simulink model "Computer"  (R2023a)
settings: Solver=VariableStepDiscrete  StartTime=0.0  StopTime=inf  RelTol=1e-3  EnableMultiTasking=on
values from neighbouring files (symbols this model uses):
  RomCode = Preprocessor(RomCode, c)    [ROM.m]
undefined symbols (not defined in the file or in its folder): c, in, RomCodeBreakpoints, RomData, RomDataBreakpoints, UartDataRx, UartDataRx_Active
libraries: Miscellaneous x281, simulink_extras x66, Memory_Blocks_Lib x46, simulink x42, Word_Multiplexers_Lib x31, Decoders_Lib x30, Encoders_Lib x10, Counters_Lib x9, Bit_Multiplexers_Lib x8, Arithmetic_Operations_Lib x5, Bit_Demultiplexers_Lib x4, Garbage x1
(part 3 of 6)

== system Computer/<0x0000..0x0FFF> ==
  note: Address_Select
  b15 : Inport
  b14 : Inport  Port=2
  b13 : Inport  Port=3
  b12 : Inport  Port=4
  b11 : Inport  Port=5
  b10 : Inport  Port=6
  b09 : Inport  Port=7
  b08 : Inport  Port=8
  b07 : Inport  Port=9
  b06 : Inport  Port=10
  b05 : Inport  Port=11
  b04 : Inport  Port=12
  b03 : Inport  Port=13
  b02 : Inport  Port=14
  b01 : Inport  Port=15
  b00 : Inport  Port=16
  1 : Constant  OutDataTypeStr=boolean
  Logical Operator{10..12,17} (4 alike) : Logic  Operator=NOT  Inputs=1  IconShape=distinctive  AllPortsSameDT=off  OutDataTypeStr=boolean
  Logical Operator9 : Logic  Inputs=16  IconShape=distinctive  AllPortsSameDT=off  OutDataTypeStr=boolean
  Terminator{1..12} (12 alike) : Terminator
  Sel(1b) : Outport
  wires:
  Logical Operator9/1 -> Sel(1b)/1
  b13/1 -> Logical Operator12/1
  b15/1 -> Logical Operator10/1
  b14/1 -> Logical Operator11/1
  b12/1 -> Logical Operator17/1
  Logical Operator10/1 -> Logical Operator9/1
  Logical Operator11/1 -> Logical Operator9/2
  Logical Operator12/1 -> Logical Operator9/3
  Logical Operator17/1 -> Logical Operator9/4
  b00/1 -> Terminator12/1
  b11/1 -> Terminator9/1
  b10/1 -> Terminator8/1
  b09/1 -> Terminator7/1
  b08/1 -> Terminator6/1
  b07/1 -> Terminator5/1
  b06/1 -> Terminator4/1
  b05/1 -> Terminator3/1
  b04/1 -> Terminator1/1
  b03/1 -> Terminator2/1
  b02/1 -> Terminator10/1
  b01/1 -> Terminator11/1
  1/1 -> Logical Operator9/16, Logical Operator9/15, Logical Operator9/14, Logical Operator9/13, Logical Operator9/12, Logical Operator9/11, Logical Operator9/10, Logical Operator9/9, Logical Operator9/8, Logical Operator9/7, Logical Operator9/6, Logical Operator9/5

== system Computer/<0x1000..0x1FFF> ==
  note: Address_Select
  b15 : Inport
  b14 : Inport  Port=2
  b13 : Inport  Port=3
  b12 : Inport  Port=4
  b11 : Inport  Port=5
  b10 : Inport  Port=6
  b09 : Inport  Port=7
  b08 : Inport  Port=8
  b07 : Inport  Port=9
  b06 : Inport  Port=10
  b05 : Inport  Port=11
  b04 : Inport  Port=12
  b03 : Inport  Port=13
  b02 : Inport  Port=14
  b01 : Inport  Port=15
  b00 : Inport  Port=16
  1 : Constant  OutDataTypeStr=boolean
  Logical Operator10 : Logic  Operator=NOT  Inputs=1  IconShape=distinctive  AllPortsSameDT=off  OutDataTypeStr=boolean
  Logical Operator11 : Logic  Operator=NOT  Inputs=1  IconShape=distinctive  AllPortsSameDT=off  OutDataTypeStr=boolean
  Logical Operator12 : Logic  Operator=NOT  Inputs=1  IconShape=distinctive  AllPortsSameDT=off  OutDataTypeStr=boolean
  Logical Operator9 : Logic  Inputs=16  IconShape=distinctive  AllPortsSameDT=off  OutDataTypeStr=boolean
  Terminator{1..13} (13 alike) : Terminator
  Sel(1b) : Outport
  wires:
  Logical Operator9/1 -> Sel(1b)/1
  b13/1 -> Logical Operator12/1
  b15/1 -> Logical Operator10/1
  b14/1 -> Logical Operator11/1
  Logical Operator10/1 -> Logical Operator9/1
  Logical Operator11/1 -> Logical Operator9/2
  Logical Operator12/1 -> Logical Operator9/3
  b00/1 -> Terminator12/1
  b11/1 -> Terminator9/1
  b10/1 -> Terminator8/1
  b09/1 -> Terminator7/1
  b08/1 -> Terminator6/1
  b07/1 -> Terminator5/1
  b06/1 -> Terminator4/1
  b05/1 -> Terminator3/1
  b04/1 -> Terminator1/1
  b03/1 -> Terminator2/1
  b02/1 -> Terminator10/1
  b01/1 -> Terminator11/1
  1/1 -> Logical Operator9/16, Logical Operator9/15, Logical Operator9/14, Logical Operator9/13, Logical Operator9/12, Logical Operator9/11, Logical Operator9/10, Logical Operator9/9, Logical Operator9/8, Logical Operator9/7, Logical Operator9/6, Logical Operator9/4, Logical Operator9/5
  b12/1 -> Terminator13/1

== system Computer/<0x2000..0x23FF> ==
  note: Address_Select
  b15 : Inport
  b14 : Inport  Port=2
  b13 : Inport  Port=3
  b12 : Inport  Port=4
  b11 : Inport  Port=5
  b10 : Inport  Port=6
  b09 : Inport  Port=7
  b08 : Inport  Port=8
  b07 : Inport  Port=9
  b06 : Inport  Port=10
  b05 : Inport  Port=11
  b04 : Inport  Port=12
  b03 : Inport  Port=13
  b02 : Inport  Port=14
  b01 : Inport  Port=15
  b00 : Inport  Port=16
  1 : Constant  OutDataTypeStr=boolean
  Logical Operator{1,4..5,10..11} (5 alike) : Logic  Operator=NOT  Inputs=1  IconShape=distinctive  AllPortsSameDT=off  OutDataTypeStr=boolean
  Logical Operator9 : Logic  Inputs=16  IconShape=distinctive  AllPortsSameDT=off  OutDataTypeStr=boolean
  Terminator{1..7,10..12} (10 alike) : Terminator
  Sel(1b) : Outport
  wires:
  Logical Operator9/1 -> Sel(1b)/1
  b15/1 -> Logical Operator10/1
  b14/1 -> Logical Operator11/1
  Logical Operator10/1 -> Logical Operator9/1
  Logical Operator11/1 -> Logical Operator9/2
  b00/1 -> Terminator12/1
  b09/1 -> Terminator7/1
  b08/1 -> Terminator6/1
  b07/1 -> Terminator5/1
  b06/1 -> Terminator4/1
  b05/1 -> Terminator3/1
  b04/1 -> Terminator1/1
  b03/1 -> Terminator2/1
  b02/1 -> Terminator10/1
  b01/1 -> Terminator11/1
  1/1 -> Logical Operator9/16, Logical Operator9/15, Logical Operator9/14, Logical Operator9/13, Logical Operator9/12, Logical Operator9/11, Logical Operator9/10, Logical Operator9/9, Logical Operator9/8, Logical Operator9/7
  Logical Operator4/1 -> Logical Operator9/4
  Logical Operator5/1 -> Logical Operator9/6
  Logical Operator1/1 -> Logical Operator9/5
  b13/1 -> Logical Operator9/3
  b12/1 -> Logical Operator4/1
  b11/1 -> Logical Operator1/1
  b10/1 -> Logical Operator5/1

== system Computer/<0xFFF6..0xFFF6> ==
  note: Address_Select
  b15 : Inport
  b14 : Inport  Port=2
  b13 : Inport  Port=3
  b12 : Inport  Port=4
  b11 : Inport  Port=5
  b10 : Inport  Port=6
  b09 : Inport  Port=7
  b08 : Inport  Port=8
  b07 : Inport  Port=9
  b06 : Inport  Port=10
  b05 : Inport  Port=11
  b04 : Inport  Port=12
  b03 : Inport  Port=13
  b02 : Inport  Port=14
  b01 : Inport  Port=15
  b00 : Inport  Port=16
  Logical Operator17 : Logic  Operator=NOT  Inputs=1  IconShape=distinctive  AllPortsSameDT=off  OutDataTypeStr=boolean
  Logical Operator2 : Logic  Operator=NOT  Inputs=1  IconShape=distinctive  AllPortsSameDT=off  OutDataTypeStr=boolean
  Logical Operator9 : Logic  Inputs=16  IconShape=distinctive  AllPortsSameDT=off  OutDataTypeStr=boolean
  Sel(1b) : Outport
  wires:
  Logical Operator9/1 -> Sel(1b)/1
  b00/1 -> Logical Operator17/1
  Logical Operator17/1 -> Logical Operator9/16
  b11/1 -> Logical Operator9/5
  b10/1 -> Logical Operator9/6
  b09/1 -> Logical Operator9/7
  b08/1 -> Logical Operator9/8
  b07/1 -> Logical Operator9/9
  b06/1 -> Logical Operator9/10
  b05/1 -> Logical Operator9/11
  b04/1 -> Logical Operator9/12
  b02/1 -> Logical Operator9/14
  b01/1 -> Logical Operator9/15
  b12/1 -> Logical Operator9/4
  b13/1 -> Logical Operator9/3
  b14/1 -> Logical Operator9/2
  b15/1 -> Logical Operator9/1
  Logical Operator2/1 -> Logical Operator9/13
  b03/1 -> Logical Operator2/1

== system Computer/<0xFFF7..0xFFF7> ==
  note: Address_Select
  b15 : Inport
  b14 : Inport  Port=2
  b13 : Inport  Port=3
  b12 : Inport  Port=4
  b11 : Inport  Port=5
  b10 : Inport  Port=6
  b09 : Inport  Port=7
  b08 : Inport  Port=8
  b07 : Inport  Port=9
  b06 : Inport  Port=10
  b05 : Inport  Port=11
  b04 : Inport  Port=12
  b03 : Inport  Port=13
  b02 : Inport  Port=14
  b01 : Inport  Port=15
  b00 : Inport  Port=16
  Logical Operator5 : Logic  Operator=NOT  Inputs=1  IconShape=distinctive  AllPortsSameDT=off  OutDataTypeStr=boolean
  Logical Operator9 : Logic  Inputs=16  IconShape=distinctive  AllPortsSameDT=off  OutDataTypeStr=boolean
  Sel(1b) : Outport
  wires:
  Logical Operator9/1 -> Sel(1b)/1
  Logical Operator5/1 -> Logical Operator9/13
  b03/1 -> Logical Operator5/1
  b15/1 -> Logical Operator9/1
  b14/1 -> Logical Operator9/2
  b13/1 -> Logical Operator9/3
  b12/1 -> Logical Operator9/4
  b11/1 -> Logical Operator9/5
  b10/1 -> Logical Operator9/6
  b09/1 -> Logical Operator9/7
  b08/1 -> Logical Operator9/8
  b07/1 -> Logical Operator9/9
  b06/1 -> Logical Operator9/10
  b05/1 -> Logical Operator9/11
  b04/1 -> Logical Operator9/12
  b02/1 -> Logical Operator9/14
  b01/1 -> Logical Operator9/15
  b00/1 -> Logical Operator9/16

== system Computer/<0xFFF8..0xFFFD> ==
  note: Address_Select
  b15 : Inport
  b14 : Inport  Port=2
  b13 : Inport  Port=3
  b12 : Inport  Port=4
  b11 : Inport  Port=5
  b10 : Inport  Port=6
  b09 : Inport  Port=7
  b08 : Inport  Port=8
  b07 : Inport  Port=9
  b06 : Inport  Port=10
  b05 : Inport  Port=11
  b04 : Inport  Port=12
  b03 : Inport  Port=13
  b02 : Inport  Port=14
  b01 : Inport  Port=15
  b00 : Inport  Port=16
  1 : Constant  OutDataTypeStr=boolean
  Logical Operator9 : Logic  Inputs=16  IconShape=distinctive  AllPortsSameDT=off  OutDataTypeStr=boolean
  Terminator10 : Terminator
  Terminator11 : Terminator
  Terminator12 : Terminator
  Sel(1b) : Outport
  wires:
  Logical Operator9/1 -> Sel(1b)/1
  b13/1 -> Logical Operator9/3
  b15/1 -> Logical Operator9/1
  b14/1 -> Logical Operator9/2
  b00/1 -> Terminator12/1
  b11/1 -> Logical Operator9/5
  b10/1 -> Logical Operator9/6
  b09/1 -> Logical Operator9/7
  b08/1 -> Logical Operator9/8
  b07/1 -> Logical Operator9/9
  b06/1 -> Logical Operator9/10
  b05/1 -> Logical Operator9/11
  b04/1 -> Logical Operator9/12
  b03/1 -> Logical Operator9/13
  b02/1 -> Terminator10/1
  b01/1 -> Terminator11/1
  1/1 -> Logical Operator9/16, Logical Operator9/15, Logical Operator9/14
  b12/1 -> Logical Operator9/4

== system Computer/<0xFFF8..0xFFFD>1 ==
  note: Address_Select
  b15 : Inport
  b14 : Inport  Port=2
  b13 : Inport  Port=3
  b12 : Inport  Port=4
  b11 : Inport  Port=5
  b10 : Inport  Port=6
  b09 : Inport  Port=7
  b08 : Inport  Port=8
  b07 : Inport  Port=9
  b06 : Inport  Port=10
  b05 : Inport  Port=11
  b04 : Inport  Port=12
  b03 : Inport  Port=13
  b02 : Inport  Port=14
  b01 : Inport  Port=15
  b00 : Inport  Port=16
  1 : Constant  OutDataTypeStr=boolean
  Logical Operator9 : Logic  Inputs=16  IconShape=distinctive  AllPortsSameDT=off  OutDataTypeStr=boolean
  Terminator10 : Terminator
  Terminator11 : Terminator
  Terminator12 : Terminator
  Sel(1b) : Outport
  wires:
  Logical Operator9/1 -> Sel(1b)/1
  b13/1 -> Logical Operator9/3
  b15/1 -> Logical Operator9/1
  b14/1 -> Logical Operator9/2
  b00/1 -> Terminator12/1
  b11/1 -> Logical Operator9/5
  b10/1 -> Logical Operator9/6
  b09/1 -> Logical Operator9/7
  b08/1 -> Logical Operator9/8
  b07/1 -> Logical Operator9/9
  b06/1 -> Logical Operator9/10
  b05/1 -> Logical Operator9/11
  b04/1 -> Logical Operator9/12
  b03/1 -> Logical Operator9/13
  b02/1 -> Terminator10/1
  b01/1 -> Terminator11/1
  1/1 -> Logical Operator9/16, Logical Operator9/15, Logical Operator9/14
  b12/1 -> Logical Operator9/4

== system Computer/<0xFFFE..0xFFFE> ==
  note: Address_Select
  b15 : Inport
  b14 : Inport  Port=2
  b13 : Inport  Port=3
  b12 : Inport  Port=4
  b11 : Inport  Port=5
  b10 : Inport  Port=6
  b09 : Inport  Port=7
  b08 : Inport  Port=8
  b07 : Inport  Port=9
  b06 : Inport  Port=10
  b05 : Inport  Port=11
  b04 : Inport  Port=12
  b03 : Inport  Port=13
  b02 : Inport  Port=14
  b01 : Inport  Port=15
  b00 : Inport  Port=16
  Logical Operator17 : Logic  Operator=NOT  Inputs=1  IconShape=distinctive  AllPortsSameDT=off  OutDataTypeStr=boolean
  Logical Operator9 : Logic  Inputs=16  IconShape=distinctive  AllPortsSameDT=off  OutDataTypeStr=boolean
  Sel(1b) : Outport
  wires:
  Logical Operator9/1 -> Sel(1b)/1
  b00/1 -> Logical Operator17/1
  Logical Operator17/1 -> Logical Operator9/16
  b11/1 -> Logical Operator9/5
  b10/1 -> Logical Operator9/6
  b09/1 -> Logical Operator9/7
  b08/1 -> Logical Operator9/8
  b07/1 -> Logical Operator9/9
  b06/1 -> Logical Operator9/10
  b05/1 -> Logical Operator9/11
  b04/1 -> Logical Operator9/12
  b03/1 -> Logical Operator9/13
  b02/1 -> Logical Operator9/14
  b01/1 -> Logical Operator9/15
  b12/1 -> Logical Operator9/4
  b13/1 -> Logical Operator9/3
  b14/1 -> Logical Operator9/2
  b15/1 -> Logical Operator9/1

== system Computer/<0xFFFF..0xFFFF> ==
  note: Address_Select
  b15 : Inport
  b14 : Inport  Port=2
  b13 : Inport  Port=3
  b12 : Inport  Port=4
  b11 : Inport  Port=5
  b10 : Inport  Port=6
  b09 : Inport  Port=7
  b08 : Inport  Port=8
  b07 : Inport  Port=9
  b06 : Inport  Port=10
  b05 : Inport  Port=11
  b04 : Inport  Port=12
  b03 : Inport  Port=13
  b02 : Inport  Port=14
  b01 : Inport  Port=15
  b00 : Inport  Port=16
  Logical Operator9 : Logic  Inputs=16  IconShape=distinctive  AllPortsSameDT=off  OutDataTypeStr=boolean
  Sel(1b) : Outport
  wires:
  Logical Operator9/1 -> Sel(1b)/1
  b13/1 -> Logical Operator9/3
  b15/1 -> Logical Operator9/1
  b14/1 -> Logical Operator9/2
  b11/1 -> Logical Operator9/5
  b10/1 -> Logical Operator9/6
  b09/1 -> Logical Operator9/7
  b08/1 -> Logical Operator9/8
  b07/1 -> Logical Operator9/9
  b06/1 -> Logical Operator9/10
  b05/1 -> Logical Operator9/11
  b04/1 -> Logical Operator9/12
  b03/1 -> Logical Operator9/13
  b12/1 -> Logical Operator9/4
  b02/1 -> Logical Operator9/14
  b01/1 -> Logical Operator9/15
  b00/1 -> Logical Operator9/16

== system Computer/<0xFFFF..0xFFFF>1 ==
  note: Address_Select
  b15 : Inport
  b14 : Inport  Port=2
  b13 : Inport  Port=3
  b12 : Inport  Port=4
  b11 : Inport  Port=5
  b10 : Inport  Port=6
  b09 : Inport  Port=7
  b08 : Inport  Port=8
  b07 : Inport  Port=9
  b06 : Inport  Port=10
  b05 : Inport  Port=11
  b04 : Inport  Port=12
  b03 : Inport  Port=13
  b02 : Inport  Port=14
  b01 : Inport  Port=15
  b00 : Inport  Port=16
  Logical Operator9 : Logic  Inputs=16  IconShape=distinctive  AllPortsSameDT=off  OutDataTypeStr=boolean
  Sel(1b) : Outport
  wires:
  Logical Operator9/1 -> Sel(1b)/1
  b13/1 -> Logical Operator9/3
  b15/1 -> Logical Operator9/1
  b14/1 -> Logical Operator9/2
  b11/1 -> Logical Operator9/5
  b10/1 -> Logical Operator9/6
  b09/1 -> Logical Operator9/7
  b08/1 -> Logical Operator9/8
  b07/1 -> Logical Operator9/9
  b06/1 -> Logical Operator9/10
  b05/1 -> Logical Operator9/11
  b04/1 -> Logical Operator9/12
  b03/1 -> Logical Operator9/13
  b12/1 -> Logical Operator9/4
  b02/1 -> Logical Operator9/14
  b01/1 -> Logical Operator9/15
  b00/1 -> Logical Operator9/16

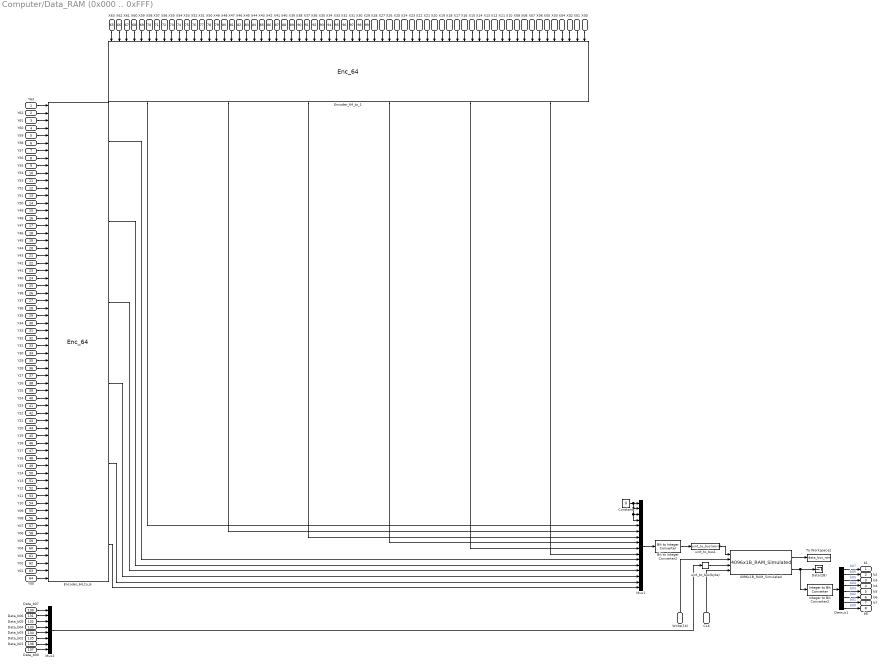
== system Computer/Data_RAM (0x000 .. 0xFFF) ==
  Y63 : Inport
  Y62 : Inport  Port=2
  Y61 : Inport  Port=3
  Y60 : Inport  Port=4
  Y59 : Inport  Port=5
  Y58 : Inport  Port=6
  Y57 : Inport  Port=7
  Y56 : Inport  Port=8
  Y55 : Inport  Port=9
  Y54 : Inport  Port=10
  Y53 : Inport  Port=11
  Y52 : Inport  Port=12
  Y51 : Inport  Port=13
  Y50 : Inport  Port=14
  Y49 : Inport  Port=15
  Y48 : Inport  Port=16
  Y47 : Inport  Port=17
  Y46 : Inport  Port=18
  Y45 : Inport  Port=19
  Y44 : Inport  Port=20
  Y43 : Inport  Port=21
  Y42 : Inport  Port=22
  Y41 : Inport  Port=23
  Y40 : Inport  Port=24
  Y39 : Inport  Port=25
  Y38 : Inport  Port=26
  Y37 : Inport  Port=27
  Y36 : Inport  Port=28
  Y35 : Inport  Port=29
  Y34 : Inport  Port=30
  Y33 : Inport  Port=31
  Y32 : Inport  Port=32
  Y31 : Inport  Port=33
  Y30 : Inport  Port=34
  Y29 : Inport  Port=35
  Y28 : Inport  Port=36
  Y27 : Inport  Port=37
  Y26 : Inport  Port=38
  Y25 : Inport  Port=39
  Y24 : Inport  Port=40
  Y23 : Inport  Port=41
  Y22 : Inport  Port=42
  Y21 : Inport  Port=43
  Y20 : Inport  Port=44
  Y19 : Inport  Port=45
  Y18 : Inport  Port=46
  Y17 : Inport  Port=47
  Y16 : Inport  Port=48
  Y15 : Inport  Port=49
  Y14 : Inport  Port=50
  Y13 : Inport  Port=51
  Y12 : Inport  Port=52
  Y11 : Inport  Port=53
  Y10 : Inport  Port=54
  Y09 : Inport  Port=55
  Y08 : Inport  Port=56
  Y07 : Inport  Port=57
  Y06 : Inport  Port=58
  Y05 : Inport  Port=59
  Y04 : Inport  Port=60
  Y03 : Inport  Port=61
  Y02 : Inport  Port=62
  Y01 : Inport  Port=63
  Y00 : Inport  Port=64
  X63 : Inport  Port=65
  X62 : Inport  Port=66
  X61 : Inport  Port=67
  X60 : Inport  Port=68
  X59 : Inport  Port=69
  X58 : Inport  Port=70
  X57 : Inport  Port=71
  X56 : Inport  Port=72
  X55 : Inport  Port=73
  X54 : Inport  Port=74
  X53 : Inport  Port=75
  X52 : Inport  Port=76
  X51 : Inport  Port=77
  X50 : Inport  Port=78
  X49 : Inport  Port=79
  X48 : Inport  Port=80
  X47 : Inport  Port=81
  X46 : Inport  Port=82
  X45 : Inport  Port=83
  X44 : Inport  Port=84
  X43 : Inport  Port=85
  X42 : Inport  Port=86
  X41 : Inport  Port=87
  X40 : Inport  Port=88
  X39 : Inport  Port=89
  X38 : Inport  Port=90
  X37 : Inport  Port=91
  X36 : Inport  Port=92
  X35 : Inport  Port=93
  X34 : Inport  Port=94
  X33 : Inport  Port=95
  X32 : Inport  Port=96
  X31 : Inport  Port=97
  X30 : Inport  Port=98
  X29 : Inport  Port=99
  X28 : Inport  Port=100
  X27 : Inport  Port=101
  X26 : Inport  Port=102
  X25 : Inport  Port=103
  X24 : Inport  Port=104
  X23 : Inport  Port=105
  X22 : Inport  Port=106
  X21 : Inport  Port=107
  X20 : Inport  Port=108
  X19 : Inport  Port=109
  X18 : Inport  Port=110
  X17 : Inport  Port=111
  X16 : Inport  Port=112
  X15 : Inport  Port=113
  X14 : Inport  Port=114
  X13 : Inport  Port=115
  X12 : Inport  Port=116
  X11 : Inport  Port=117
  X10 : Inport  Port=118
  X09 : Inport  Port=119
  X08 : Inport  Port=120
  X07 : Inport  Port=121
  X06 : Inport  Port=122
  X05 : Inport  Port=123
  X03 : Inport  Port=124
  X04 : Inport  Port=125
  X02 : Inport  Port=126
  X01 : Inport  Port=127
  X00 : Inport  Port=128
  CLK : Inport  Port=129
  Data_b07 : Inport  Port=130
  Data_b06 : Inport  Port=131
  Data_b05 : Inport  Port=132
  Data_b04 : Inport  Port=133
  Data_b03 : Inport  Port=134
  Data_b02 : Inport  Port=135
  Data_b01 : Inport  Port=136
  Data_b00 : Inport  Port=137
  Write(1b) : Inport  Port=138
  4096x1B_RAM_Simulated : Memory_Blocks_Lib/4096x1B_RAM_Simulated  SystemSampleTime=-1  VariantActivationTime=update diagram  Latency=0  AutoFrameSizeCalculation=off
      settings: LibrarySourceBlock=Memory_Blocks_Lib/Memory_Blocks_Lib/4096x1B_RAM_Simulated
  Bit to Integer Converter2 : simulink/Logic and Bit Operations/Bit to Integer Converter  nbits=16  bitOrder=MSB first  signedOutputValues=Unsigned  outDtype=uint16  outDtypeSigned=Inherit via internal rule
      settings: LibrarySourceBlock=|
      | commutil2/Bit to Integer
      | Converter
  Constant : Constant  Value=0  OutDataTypeStr=boolean
  Data(2B) : Terminator
  Demux1 : Demux  Outputs=8
  Encoder_64_to_1 : Encoders_Lib/Enc_64  SystemSampleTime=-1  VariantActivationTime=update diagram  Latency=0  AutoFrameSizeCalculation=off
      settings: LibrarySourceBlock=Garbage/Encoder_64_to_6
  Encoder_64_to_6 : Encoders_Lib/Enc_64  SystemSampleTime=-1  VariantActivationTime=update diagram  Latency=0  AutoFrameSizeCalculation=off
      settings: LibrarySourceBlock=Garbage/Encoder_64_to_6
  Integer to Bit Converter2 : simulink/Logic and Bit Operations/Integer to Bit Converter  nbits=16  signedInputValues=Unsigned  bitOrder=MSB first  outDtype=boolean
      settings: LibrarySourceBlock=|
      | commutil2/Integer to Bit
      | Converter
  Mux1 : Mux  Inputs=16
  Mux2 : Mux  Inputs=8
  To Workspace2 : ToWorkspace  VariableName=data_bus_ram  SampleTime=-1
      settings: MaxDataPoints=1  Save2DSignal=2-D array (concatenate along first dimension)
  uint_to_bus(byte) : Miscellaneous/uint_to_bus(byte)  SystemSampleTime=-1  VariantActivationTime=update diagram  Latency=0  AutoFrameSizeCalculation=off
  uint_to_bus1 : Miscellaneous/uint_to_bus(word)
      settings: LibrarySourceBlock=Miscellaneous/uint_to_bus
  b1 : Outport
  b2 : Outport  Port=2
  b3 : Outport  Port=3
  b4 : Outport  Port=4
  b5 : Outport  Port=5
  b6 : Outport  Port=6
  b7 : Outport  Port=7
  b8 : Outport  Port=8
  wires:
  Y04/1 -> Encoder_64_to_6/60
  Y02/1 -> Encoder_64_to_6/62
  Y57/1 -> Encoder_64_to_6/7
  Y07/1 -> Encoder_64_to_6/57
  Y22/1 -> Encoder_64_to_6/42
  Y33/1 -> Encoder_64_to_6/31
  Y54/1 -> Encoder_64_to_6/10
  Y52/1 -> Encoder_64_to_6/12
  Y39/1 -> Encoder_64_to_6/25
  Y19/1 -> Encoder_64_to_6/45
  Y60/1 -> Encoder_64_to_6/4
  Y12/1 -> Encoder_64_to_6/52
  Y44/1 -> Encoder_64_to_6/20
  Y51/1 -> Encoder_64_to_6/13
  Y58/1 -> Encoder_64_to_6/6
  Y16/1 -> Encoder_64_to_6/48
  Y11/1 -> Encoder_64_to_6/53
  Y61/1 -> Encoder_64_to_6/3
  Y32/1 -> Encoder_64_to_6/32
  Y29/1 -> Encoder_64_to_6/35
  Y15/1 -> Encoder_64_to_6/49
  Y21/1 -> Encoder_64_to_6/43
  Y03/1 -> Encoder_64_to_6/61
  Y00/1 -> Encoder_64_to_6/64
  Y23/1 -> Encoder_64_to_6/41
  Y38/1 -> Encoder_64_to_6/26
  Y05/1 -> Encoder_64_to_6/59
  Y01/1 -> Encoder_64_to_6/63
  Y06/1 -> Encoder_64_to_6/58
  Y34/1 -> Encoder_64_to_6/30
  Y08/1 -> Encoder_64_to_6/56
  Y25/1 -> Encoder_64_to_6/39
  Y36/1 -> Encoder_64_to_6/28
  Y59/1 -> Encoder_64_to_6/5
  Y40/1 -> Encoder_64_to_6/24
  Y09/1 -> Encoder_64_to_6/55
  Y42/1 -> Encoder_64_to_6/22
  Y24/1 -> Encoder_64_to_6/40
  Y62/1 -> Encoder_64_to_6/2
  Y30/1 -> Encoder_64_to_6/34
  Y53/1 -> Encoder_64_to_6/11
  Y41/1 -> Encoder_64_to_6/23
  Y35/1 -> Encoder_64_to_6/29
  Y63/1 -> Encoder_64_to_6/1
  Y48/1 -> Encoder_64_to_6/16
  Y55/1 -> Encoder_64_to_6/9
  Y13/1 -> Encoder_64_to_6/51
  Y37/1 -> Encoder_64_to_6/27
  Y45/1 -> Encoder_64_to_6/19
  Y43/1 -> Encoder_64_to_6/21
  Y50/1 -> Encoder_64_to_6/14
  Y27/1 -> Encoder_64_to_6/37
  Y49/1 -> Encoder_64_to_6/15
  Y14/1 -> Encoder_64_to_6/50
  Y18/1 -> Encoder_64_to_6/46
  Y56/1 -> Encoder_64_to_6/8
  Y26/1 -> Encoder_64_to_6/38
  Y31/1 -> Encoder_64_to_6/33
  Y20/1 -> Encoder_64_to_6/44
  Y10/1 -> Encoder_64_to_6/54
  Y17/1 -> Encoder_64_to_6/47
  Y28/1 -> Encoder_64_to_6/36
  Y47/1 -> Encoder_64_to_6/17
  Y46/1 -> Encoder_64_to_6/18
  X63/1 -> Encoder_64_to_1/1
  X62/1 -> Encoder_64_to_1/2
  X61/1 -> Encoder_64_to_1/3
  X60/1 -> Encoder_64_to_1/4
  X59/1 -> Encoder_64_to_1/5
  X58/1 -> Encoder_64_to_1/6
  X57/1 -> Encoder_64_to_1/7
  X56/1 -> Encoder_64_to_1/8
  X55/1 -> Encoder_64_to_1/9
  X54/1 -> Encoder_64_to_1/10
  X53/1 -> Encoder_64_to_1/11
  X52/1 -> Encoder_64_to_1/12
  X51/1 -> Encoder_64_to_1/13
  X50/1 -> Encoder_64_to_1/14
  X49/1 -> Encoder_64_to_1/15
  X48/1 -> Encoder_64_to_1/16
  X47/1 -> Encoder_64_to_1/17
  X46/1 -> Encoder_64_to_1/18
  X45/1 -> Encoder_64_to_1/19
  X44/1 -> Encoder_64_to_1/20
  X43/1 -> Encoder_64_to_1/21
  X42/1 -> Encoder_64_to_1/22
  X41/1 -> Encoder_64_to_1/23
  X40/1 -> Encoder_64_to_1/24
  X39/1 -> Encoder_64_to_1/25
  X38/1 -> Encoder_64_to_1/26
  X37/1 -> Encoder_64_to_1/27
  X36/1 -> Encoder_64_to_1/28
  X35/1 -> Encoder_64_to_1/29
  X34/1 -> Encoder_64_to_1/30
  X33/1 -> Encoder_64_to_1/31
  X32/1 -> Encoder_64_to_1/32
  X31/1 -> Encoder_64_to_1/33
  X30/1 -> Encoder_64_to_1/34
  X29/1 -> Encoder_64_to_1/35
  X28/1 -> Encoder_64_to_1/36
  X27/1 -> Encoder_64_to_1/37
  X26/1 -> Encoder_64_to_1/38
  X25/1 -> Encoder_64_to_1/39
  X24/1 -> Encoder_64_to_1/40
  X23/1 -> Encoder_64_to_1/41
  X22/1 -> Encoder_64_to_1/42
  X21/1 -> Encoder_64_to_1/43
  X20/1 -> Encoder_64_to_1/44
  X19/1 -> Encoder_64_to_1/45
  X18/1 -> Encoder_64_to_1/46
  X17/1 -> Encoder_64_to_1/47
  X16/1 -> Encoder_64_to_1/48
  X15/1 -> Encoder_64_to_1/49
  X14/1 -> Encoder_64_to_1/50
  X13/1 -> Encoder_64_to_1/51
  X12/1 -> Encoder_64_to_1/52
  X11/1 -> Encoder_64_to_1/53
  X10/1 -> Encoder_64_to_1/54
  X09/1 -> Encoder_64_to_1/55
  X08/1 -> Encoder_64_to_1/56
  X07/1 -> Encoder_64_to_1/57
  X06/1 -> Encoder_64_to_1/58
  X05/1 -> Encoder_64_to_1/59
  X04/1 -> Encoder_64_to_1/61
  X03/1 -> Encoder_64_to_1/60
  X02/1 -> Encoder_64_to_1/62
  X01/1 -> Encoder_64_to_1/63
  X00/1 -> Encoder_64_to_1/64
  Bit to Integer Converter2/1 -> uint_to_bus1/1
  Write(1b)/1 -> 4096x1B_RAM_Simulated/2
  4096x1B_RAM_Simulated/1 -> To Workspace2/1
  Constant/1 -> Mux1/2, Mux1/3, Mux1/4, Mux1/1
  CLK/1 -> 4096x1B_RAM_Simulated/4
  Mux2/1 -> uint_to_bus(byte)/1
  Mux1/1 -> Bit to Integer Converter2/1
  uint_to_bus1/1 -> 4096x1B_RAM_Simulated/1
  Encoder_64_to_6/6 -> Mux1/16
  Encoder_64_to_6/5 -> Mux1/15
  Encoder_64_to_6/4 -> Mux1/14
  Encoder_64_to_6/3 -> Mux1/13
  Encoder_64_to_6/2 -> Mux1/12
  Encoder_64_to_6/1 -> Mux1/11
  Encoder_64_to_1/6 -> Mux1/10
  Encoder_64_to_1/5 -> Mux1/9
  Encoder_64_to_1/4 -> Mux1/8
  Encoder_64_to_1/3 -> Mux1/7
  Encoder_64_to_1/2 -> Mux1/6
  Encoder_64_to_1/1 -> Mux1/5
  4096x1B_RAM_Simulated/2 -> Data(2B)/1, Integer to Bit Converter2/1
  uint_to_bus(byte)/1 -> 4096x1B_RAM_Simulated/3
  Data_b07/1 -> Mux2/1
  Data_b06/1 -> Mux2/2
  Data_b05/1 -> Mux2/3
  Data_b04/1 -> Mux2/4
  Data_b03/1 -> Mux2/5
  Data_b02/1 -> Mux2/6
  Data_b01/1 -> Mux2/7
  Data_b00/1 -> Mux2/8
  Demux1/5 -> b5/1  "b03"
  Demux1/8 -> b8/1  "b00"
  Demux1/3 -> b3/1  "b05"
  Demux1/2 -> b2/1  "b06"
  Demux1/1 -> b1/1  "b07"
  Demux1/7 -> b7/1  "b01"
  Demux1/6 -> b6/1  "b02"
  Demux1/4 -> b4/1  "b04"
  Integer to Bit Converter2/1 -> Demux1/1

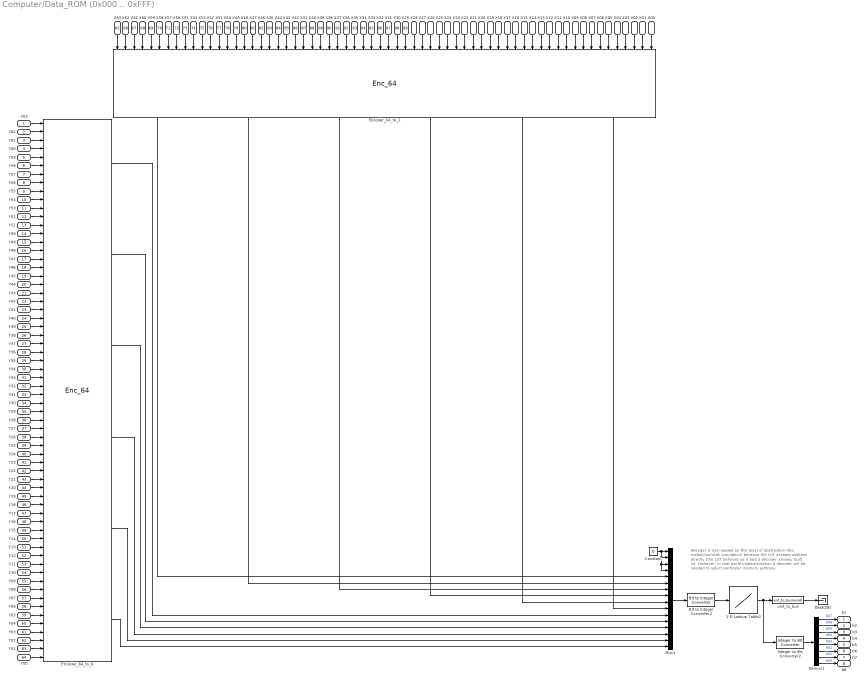
== system Computer/Data_ROM (0x000 .. 0xFFF) ==
  note: Decoder is not needed on this level of abstraction (the matlab/simulink simulation) because the LUT accepts address directly (the LUT behaves as it had a decoder already built in). However, in real-world implementation a decoder will be needed to select particular memory address.
  Y63 : Inport
  Y62 : Inport  Port=2
  Y61 : Inport  Port=3
  Y60 : Inport  Port=4
  Y59 : Inport  Port=5
  Y58 : Inport  Port=6
  Y57 : Inport  Port=7
  Y56 : Inport  Port=8
  Y55 : Inport  Port=9
  Y54 : Inport  Port=10
  Y53 : Inport  Port=11
  Y52 : Inport  Port=12
  Y51 : Inport  Port=13
  Y50 : Inport  Port=14
  Y49 : Inport  Port=15
  Y48 : Inport  Port=16
  Y47 : Inport  Port=17
  Y46 : Inport  Port=18
  Y45 : Inport  Port=19
  Y44 : Inport  Port=20
  Y43 : Inport  Port=21
  Y42 : Inport  Port=22
  Y41 : Inport  Port=23
  Y40 : Inport  Port=24
  Y39 : Inport  Port=25
  Y38 : Inport  Port=26
  Y37 : Inport  Port=27
  Y36 : Inport  Port=28
  Y35 : Inport  Port=29
  Y34 : Inport  Port=30
  Y33 : Inport  Port=31
  Y32 : Inport  Port=32
  Y31 : Inport  Port=33
  Y30 : Inport  Port=34
  Y29 : Inport  Port=35
  Y28 : Inport  Port=36
  Y27 : Inport  Port=37
  Y26 : Inport  Port=38
  Y25 : Inport  Port=39
  Y24 : Inport  Port=40
  Y23 : Inport  Port=41
  Y22 : Inport  Port=42
  Y21 : Inport  Port=43
  Y20 : Inport  Port=44
  Y19 : Inport  Port=45
  Y18 : Inport  Port=46
  Y17 : Inport  Port=47
  Y16 : Inport  Port=48
  Y15 : Inport  Port=49
  Y14 : Inport  Port=50
  Y13 : Inport  Port=51
  Y12 : Inport  Port=52
  Y11 : Inport  Port=53
  Y10 : Inport  Port=54
  Y09 : Inport  Port=55
  Y08 : Inport  Port=56
  Y07 : Inport  Port=57
  Y06 : Inport  Port=58
  Y05 : Inport  Port=59
  Y04 : Inport  Port=60
  Y03 : Inport  Port=61
  Y02 : Inport  Port=62
  Y01 : Inport  Port=63
  Y00 : Inport  Port=64
  X63 : Inport  Port=65
  X62 : Inport  Port=66
  X61 : Inport  Port=67
  X60 : Inport  Port=68
  X59 : Inport  Port=69
  X58 : Inport  Port=70
  X57 : Inport  Port=71
  X56 : Inport  Port=72
  X55 : Inport  Port=73
  X54 : Inport  Port=74
  X53 : Inport  Port=75
  X52 : Inport  Port=76
  X51 : Inport  Port=77
  X50 : Inport  Port=78
  X49 : Inport  Port=79
  X48 : Inport  Port=80
  X47 : Inport  Port=81
  X46 : Inport  Port=82
  X45 : Inport  Port=83
  X44 : Inport  Port=84
  X43 : Inport  Port=85
  X42 : Inport  Port=86
  X41 : Inport  Port=87
  X40 : Inport  Port=88
  X39 : Inport  Port=89
  X38 : Inport  Port=90
  X37 : Inport  Port=91
  X36 : Inport  Port=92
  X35 : Inport  Port=93
  X34 : Inport  Port=94
  X33 : Inport  Port=95
  X32 : Inport  Port=96
  X31 : Inport  Port=97
  X30 : Inport  Port=98
  X29 : Inport  Port=99
  X28 : Inport  Port=100
  X27 : Inport  Port=101
  X26 : Inport  Port=102
  X25 : Inport  Port=103
  X24 : Inport  Port=104
  X23 : Inport  Port=105
  X22 : Inport  Port=106
  X21 : Inport  Port=107
  X20 : Inport  Port=108
  X19 : Inport  Port=109
  X18 : Inport  Port=110
  X17 : Inport  Port=111
  X16 : Inport  Port=112
  X15 : Inport  Port=113
  X14 : Inport  Port=114
  X13 : Inport  Port=115
  X12 : Inport  Port=116
  X11 : Inport  Port=117
  X10 : Inport  Port=118
  X09 : Inport  Port=119
  X08 : Inport  Port=120
  X07 : Inport  Port=121
  X06 : Inport  Port=122
  X05 : Inport  Port=123
  X04 : Inport  Port=124
  X03 : Inport  Port=125
  X02 : Inport  Port=126
  X01 : Inport  Port=127
  X00 : Inport  Port=128
  1-D Lookup Table2 : Lookup_n-D  NumberOfTableDimensions=1  BreakpointsForDimension1=RomDataBreakpoints  Table=RomData  InterpMethod=Flat  InternalRulePriority=Speed  RndMeth=Simplest
  Bit to Integer Converter2 : simulink/Logic and Bit Operations/Bit to Integer Converter  nbits=16  bitOrder=MSB first  signedOutputValues=Unsigned  outDtype=uint16  outDtypeSigned=Inherit via internal rule
      settings: LibrarySourceBlock=|
      | commutil2/Bit to Integer
      | Converter
  Constant : Constant  Value=0  OutDataTypeStr=boolean
  Data(2B) : Terminator
  Demux1 : Demux  Outputs=8
  Encoder_64_to_1 : Encoders_Lib/Enc_64  SystemSampleTime=-1  VariantActivationTime=update diagram  Latency=0  AutoFrameSizeCalculation=off
      settings: LibrarySourceBlock=Garbage/Encoder_64_to_6
  Encoder_64_to_6 : Encoders_Lib/Enc_64  SystemSampleTime=-1  VariantActivationTime=update diagram  Latency=0  AutoFrameSizeCalculation=off
      settings: LibrarySourceBlock=Garbage/Encoder_64_to_6
  Integer to Bit Converter2 : simulink/Logic and Bit Operations/Integer to Bit Converter  nbits=16  signedInputValues=Unsigned  bitOrder=MSB first  outDtype=boolean
      settings: LibrarySourceBlock=|
      | commutil2/Integer to Bit
      | Converter
  Mux1 : Mux  Inputs=16
  uint_to_bus : Miscellaneous/uint_to_bus(word)
      settings: LibrarySourceBlock=Miscellaneous/uint_to_bus
  b1 : Outport
  b2 : Outport  Port=2
  b3 : Outport  Port=3
  b4 : Outport  Port=4
  b5 : Outport  Port=5
  b6 : Outport  Port=6
  b7 : Outport  Port=7
  b8 : Outport  Port=8
  wires:
  Mux1/1 -> Bit to Integer Converter2/1
  uint_to_bus/1 -> Data(2B)/1
  Y04/1 -> Encoder_64_to_6/60
  Y02/1 -> Encoder_64_to_6/62
  Y57/1 -> Encoder_64_to_6/7
  Y07/1 -> Encoder_64_to_6/57
  Y22/1 -> Encoder_64_to_6/42
  Y33/1 -> Encoder_64_to_6/31
  Y54/1 -> Encoder_64_to_6/10
  Y52/1 -> Encoder_64_to_6/12
  Y39/1 -> Encoder_64_to_6/25
  Y19/1 -> Encoder_64_to_6/45
  Y60/1 -> Encoder_64_to_6/4
  Y12/1 -> Encoder_64_to_6/52
  Y44/1 -> Encoder_64_to_6/20
  Y51/1 -> Encoder_64_to_6/13
  Y58/1 -> Encoder_64_to_6/6
  Y16/1 -> Encoder_64_to_6/48
  Y11/1 -> Encoder_64_to_6/53
  Y61/1 -> Encoder_64_to_6/3
  Y32/1 -> Encoder_64_to_6/32
  Y29/1 -> Encoder_64_to_6/35
  Y15/1 -> Encoder_64_to_6/49
  Y21/1 -> Encoder_64_to_6/43
  Y03/1 -> Encoder_64_to_6/61
  Y00/1 -> Encoder_64_to_6/64
  Y23/1 -> Encoder_64_to_6/41
  Y38/1 -> Encoder_64_to_6/26
  Y05/1 -> Encoder_64_to_6/59
  Y01/1 -> Encoder_64_to_6/63
  Y06/1 -> Encoder_64_to_6/58
  Y34/1 -> Encoder_64_to_6/30
  Y08/1 -> Encoder_64_to_6/56
  Y25/1 -> Encoder_64_to_6/39
  Y36/1 -> Encoder_64_to_6/28
  Y59/1 -> Encoder_64_to_6/5
  Y40/1 -> Encoder_64_to_6/24
  Y09/1 -> Encoder_64_to_6/55
  Y42/1 -> Encoder_64_to_6/22
  Y24/1 -> Encoder_64_to_6/40
  Y62/1 -> Encoder_64_to_6/2
  Y30/1 -> Encoder_64_to_6/34
  Y53/1 -> Encoder_64_to_6/11
  Y41/1 -> Encoder_64_to_6/23
  Y35/1 -> Encoder_64_to_6/29
  Y63/1 -> Encoder_64_to_6/1
  Y48/1 -> Encoder_64_to_6/16
  Y55/1 -> Encoder_64_to_6/9
  Y13/1 -> Encoder_64_to_6/51
  Y37/1 -> Encoder_64_to_6/27
  Y45/1 -> Encoder_64_to_6/19
  Y43/1 -> Encoder_64_to_6/21
  Y50/1 -> Encoder_64_to_6/14
  Y27/1 -> Encoder_64_to_6/37
  Y49/1 -> Encoder_64_to_6/15
  Y14/1 -> Encoder_64_to_6/50
  Y18/1 -> Encoder_64_to_6/46
  Y56/1 -> Encoder_64_to_6/8
  Y26/1 -> Encoder_64_to_6/38
  Y31/1 -> Encoder_64_to_6/33
  Y20/1 -> Encoder_64_to_6/44
  Y10/1 -> Encoder_64_to_6/54
  Y17/1 -> Encoder_64_to_6/47
  Y28/1 -> Encoder_64_to_6/36
  Y47/1 -> Encoder_64_to_6/17
  Y46/1 -> Encoder_64_to_6/18
  Constant/1 -> Mux1/2, Mux1/3, Mux1/4, Mux1/1
  X63/1 -> Encoder_64_to_1/1
  X62/1 -> Encoder_64_to_1/2
  X61/1 -> Encoder_64_to_1/3
  X60/1 -> Encoder_64_to_1/4
  X59/1 -> Encoder_64_to_1/5
  X58/1 -> Encoder_64_to_1/6
  X57/1 -> Encoder_64_to_1/7
  X56/1 -> Encoder_64_to_1/8
  X55/1 -> Encoder_64_to_1/9
  X54/1 -> Encoder_64_to_1/10
  X53/1 -> Encoder_64_to_1/11
  X52/1 -> Encoder_64_to_1/12
  X51/1 -> Encoder_64_to_1/13
  X50/1 -> Encoder_64_to_1/14
  X49/1 -> Encoder_64_to_1/15
  X48/1 -> Encoder_64_to_1/16
  X47/1 -> Encoder_64_to_1/17
  X46/1 -> Encoder_64_to_1/18
  X45/1 -> Encoder_64_to_1/19
  X44/1 -> Encoder_64_to_1/20
  X43/1 -> Encoder_64_to_1/21
  X42/1 -> Encoder_64_to_1/22
  X41/1 -> Encoder_64_to_1/23
  X40/1 -> Encoder_64_to_1/24
  X39/1 -> Encoder_64_to_1/25
  X38/1 -> Encoder_64_to_1/26
  X37/1 -> Encoder_64_to_1/27
  X36/1 -> Encoder_64_to_1/28
  X35/1 -> Encoder_64_to_1/29
  X34/1 -> Encoder_64_to_1/30
  X33/1 -> Encoder_64_to_1/31
  X32/1 -> Encoder_64_to_1/32
  X31/1 -> Encoder_64_to_1/33
  X30/1 -> Encoder_64_to_1/34
  X29/1 -> Encoder_64_to_1/35
  X28/1 -> Encoder_64_to_1/36
  X27/1 -> Encoder_64_to_1/37
  X26/1 -> Encoder_64_to_1/38
  X25/1 -> Encoder_64_to_1/39
  X24/1 -> Encoder_64_to_1/40
  X23/1 -> Encoder_64_to_1/41
  X22/1 -> Encoder_64_to_1/42
  X21/1 -> Encoder_64_to_1/43
  X20/1 -> Encoder_64_to_1/44
  X19/1 -> Encoder_64_to_1/45
  X18/1 -> Encoder_64_to_1/46
  X17/1 -> Encoder_64_to_1/47
  X16/1 -> Encoder_64_to_1/48
  X15/1 -> Encoder_64_to_1/49
  X14/1 -> Encoder_64_to_1/50
  X13/1 -> Encoder_64_to_1/51
  X12/1 -> Encoder_64_to_1/52
  X11/1 -> Encoder_64_to_1/53
  X10/1 -> Encoder_64_to_1/54
  X09/1 -> Encoder_64_to_1/55
  X08/1 -> Encoder_64_to_1/56
  X07/1 -> Encoder_64_to_1/57
  X06/1 -> Encoder_64_to_1/58
  X05/1 -> Encoder_64_to_1/59
  X04/1 -> Encoder_64_to_1/60
  X03/1 -> Encoder_64_to_1/61
  X02/1 -> Encoder_64_to_1/62
  X01/1 -> Encoder_64_to_1/63
  X00/1 -> Encoder_64_to_1/64
  Bit to Integer Converter2/1 -> 1-D Lookup Table2/1
  Encoder_64_to_6/6 -> Mux1/16
  Encoder_64_to_6/5 -> Mux1/15
  Encoder_64_to_6/4 -> Mux1/14
  Encoder_64_to_6/3 -> Mux1/13
  Encoder_64_to_6/2 -> Mux1/12
  Encoder_64_to_6/1 -> Mux1/11
  Encoder_64_to_1/6 -> Mux1/10
  Encoder_64_to_1/5 -> Mux1/9
  Encoder_64_to_1/4 -> Mux1/8
  Encoder_64_to_1/3 -> Mux1/7
  Encoder_64_to_1/2 -> Mux1/6
  Encoder_64_to_1/1 -> Mux1/5
  1-D Lookup Table2/1 -> Integer to Bit Converter2/1, uint_to_bus/1
  Integer to Bit Converter2/1 -> Demux1/1
  Demux1/1 -> b1/1  "b07"
  Demux1/3 -> b3/1  "b05"
  Demux1/7 -> b7/1  "b01"
  Demux1/8 -> b8/1  "b00"
  Demux1/6 -> b6/1  "b02"
  Demux1/2 -> b2/1  "b06"
  Demux1/4 -> b4/1  "b04"
  Demux1/5 -> b5/1  "b03"

== system Computer/Instruction_AND ==
  note: Word_And
  A(2B) : Inport
  B(2B) : Inport  Port=2
  Bus Creator : BusCreator  Inputs=16
  Bus Selector : BusSelector  OutputSignals=b15,b14,b13,b12,b11,b10,b09,b08,b07,b06,b05,b04,b03,b02,b01,b00
  Bus Selector1 : BusSelector  OutputSignals=b15,b14,b13,b12,b11,b10,b09,b08,b07,b06,b05,b04,b03,b02,b01,b00
  Logical Operator{8..23} (16 alike) : Logic  IconShape=distinctive  AllPortsSameDT=off  OutDataTypeStr=boolean
  A.B(2B) : Outport  OutputWhenDisabled=reset
  wires:
  Logical Operator8/1 -> Bus Creator/1  "b15"
  Logical Operator9/1 -> Bus Creator/2  "b14"
  Logical Operator16/1 -> Bus Creator/3  "b13"
  Logical Operator21/1 -> Bus Creator/8  "b08"
  Logical Operator20/1 -> Bus Creator/7  "b09"
  Logical Operator19/1 -> Bus Creator/6  "b10"
  Logical Operator17/1 -> Bus Creator/4  "b12"
  Logical Operator18/1 -> Bus Creator/5  "b11"
  Bus Selector1/8 -> Logical Operator21/2  "<b08>"
  Bus Selector/8 -> Logical Operator21/1  "<b08>"
  Bus Selector1/7 -> Logical Operator20/2  "<b09>"
  Bus Selector/7 -> Logical Operator20/1  "<b09>"
  Bus Selector1/6 -> Logical Operator19/2  "<b10>"
  Bus Selector/6 -> Logical Operator19/1  "<b10>"
  Bus Selector1/5 -> Logical Operator18/2  "<b11>"
  Bus Selector/5 -> Logical Operator18/1  "<b11>"
  Bus Selector1/4 -> Logical Operator17/2  "<b12>"
  Bus Selector/4 -> Logical Operator17/1  "<b12>"
  Bus Selector/3 -> Logical Operator16/1  "<b13>"
  Bus Selector1/3 -> Logical Operator16/2  "<b13>"
  Bus Selector1/2 -> Logical Operator9/2  "<b14>"
  Bus Selector/2 -> Logical Operator9/1  "<b14>"
  Bus Selector1/1 -> Logical Operator8/2  "<b15>"
  Bus Selector/1 -> Logical Operator8/1  "<b15>"
  Logical Operator22/1 -> Bus Creator/9  "b07"
  Logical Operator23/1 -> Bus Creator/10  "b06"
  Logical Operator10/1 -> Bus Creator/11  "b05"
  Logical Operator15/1 -> Bus Creator/16  "b00"
  Logical Operator14/1 -> Bus Creator/15  "b01"
  Logical Operator13/1 -> Bus Creator/14  "b02"
  Logical Operator11/1 -> Bus Creator/12  "b04"
  Logical Operator12/1 -> Bus Creator/13  "b03"
  Bus Selector/10 -> Logical Operator23/1  "<b06>"
  Bus Selector/9 -> Logical Operator22/1  "<b07>"
  Bus Selector/11 -> Logical Operator10/1  "<b05>"
  Bus Selector/12 -> Logical Operator11/1  "<b04>"
  Bus Selector/13 -> Logical Operator12/1  "<b03>"
  Bus Selector/14 -> Logical Operator13/1  "<b02>"
  Bus Selector/15 -> Logical Operator14/1  "<b01>"
  Bus Selector/16 -> Logical Operator15/1  "<b00>"
  Bus Selector1/9 -> Logical Operator22/2  "<b07>"
  Bus Selector1/10 -> Logical Operator23/2  "<b06>"
  Bus Selector1/11 -> Logical Operator10/2  "<b05>"
  Bus Selector1/12 -> Logical Operator11/2  "<b04>"
  Bus Selector1/13 -> Logical Operator12/2  "<b03>"
  Bus Selector1/14 -> Logical Operator13/2  "<b02>"
  Bus Selector1/15 -> Logical Operator14/2  "<b01>"
  Bus Selector1/16 -> Logical Operator15/2  "<b00>"
  Bus Creator/1 -> A.B(2B)/1
  B(2B)/1 -> Bus Selector1/1
  A(2B)/1 -> Bus Selector/1

== system Computer/Instruction_LDL ==
  note: Load_Lower_Byte
  Data_1(2B) : Inport
  Data_0(2B) : Inport  Port=2
  Bus Creator : BusCreator  Inputs=16
  Bus Selector1 : BusSelector  OutputSignals=b07,b06,b05,b04,b03,b02,b01,b00
  Bus Selector2 : BusSelector  OutputSignals=b15,b14,b13,b12,b11,b10,b09,b08
  Data(2B) : Outport  OutputWhenDisabled=reset
  wires:
  Data_0(2B)/1 -> Bus Selector1/1
  Bus Creator/1 -> Data(2B)/1
  Data_1(2B)/1 -> Bus Selector2/1
  Bus Selector2/1 -> Bus Creator/1  "<b15>"
  Bus Selector2/2 -> Bus Creator/2  "<b14>"
  Bus Selector2/3 -> Bus Creator/3  "<b13>"
  Bus Selector2/4 -> Bus Creator/4  "<b12>"
  Bus Selector2/5 -> Bus Creator/5  "<b11>"
  Bus Selector2/6 -> Bus Creator/6  "<b10>"
  Bus Selector2/7 -> Bus Creator/7  "<b09>"
  Bus Selector2/8 -> Bus Creator/8  "<b08>"
  Bus Selector1/1 -> Bus Creator/9  "<b07>"
  Bus Selector1/2 -> Bus Creator/10  "<b06>"
  Bus Selector1/3 -> Bus Creator/11  "<b05>"
  Bus Selector1/4 -> Bus Creator/12  "<b04>"
  Bus Selector1/5 -> Bus Creator/13  "<b03>"
  Bus Selector1/6 -> Bus Creator/14  "<b02>"
  Bus Selector1/7 -> Bus Creator/15  "<b01>"
  Bus Selector1/8 -> Bus Creator/16  "<b00>"

== system Computer/Instruction_LDU ==
  note: Load_Upper_Byte
  Data_0(2B) : Inport
  Data_1(2B) : Inport  Port=2
  Bus Creator : BusCreator  Inputs=16
  Bus Selector1 : BusSelector  OutputSignals=b07,b06,b05,b04,b03,b02,b01,b00
  Bus Selector2 : BusSelector  OutputSignals=b07,b06,b05,b04,b03,b02,b01,b00
  Name{1..7,16} (8 alike) : Miscellaneous/Name
  Data(2B) : Outport  OutputWhenDisabled=reset
  wires:
  Bus Creator/1 -> Data(2B)/1
  Data_1(2B)/1 -> Bus Selector1/1
  Data_0(2B)/1 -> Bus Selector2/1
  Name16/1 -> Bus Creator/1  "b15"
  Name1/1 -> Bus Creator/2  "b14"
  Name6/1 -> Bus Creator/3  "b13"
  Name2/1 -> Bus Creator/4  "b12"
  Name3/1 -> Bus Creator/5  "b11"
  Name4/1 -> Bus Creator/6  "b10"
  Name5/1 -> Bus Creator/7  "b09"
  Name7/1 -> Bus Creator/8  "b08"
  Bus Selector1/1 -> Name16/1  "<b07>"
  Bus Selector1/2 -> Name1/1  "<b06>"
  Bus Selector1/3 -> Name6/1  "<b05>"
  Bus Selector1/4 -> Name2/1  "<b04>"
  Bus Selector1/5 -> Name3/1  "<b03>"
  Bus Selector1/6 -> Name4/1  "<b02>"
  Bus Selector1/7 -> Name5/1  "<b01>"
  Bus Selector1/8 -> Name7/1  "<b00>"
  Bus Selector2/1 -> Bus Creator/9  "<b07>"
  Bus Selector2/2 -> Bus Creator/10  "<b06>"
  Bus Selector2/3 -> Bus Creator/11  "<b05>"
  Bus Selector2/4 -> Bus Creator/12  "<b04>"
  Bus Selector2/5 -> Bus Creator/13  "<b03>"
  Bus Selector2/6 -> Bus Creator/14  "<b02>"
  Bus Selector2/7 -> Bus Creator/15  "<b01>"
  Bus Selector2/8 -> Bus Creator/16  "<b00>"

== system Computer/Instruction_MOVU ==
  note: Move_Upper_Byte
  Data_1(2B) : Inport
  Data_0(2B) : Inport  Port=2
  Bus Creator3 : BusCreator  Inputs=16
  Bus Selector : BusSelector  OutputSignals=b07,b06,b05,b04,b03,b02,b01,b00
  Bus Selector1 : BusSelector  OutputSignals=b07,b06,b05,b04,b03,b02,b01,b00
  Name{1..8} (8 alike) : Miscellaneous/Name
  Data(2B) : Outport  OutputWhenDisabled=reset
  wires:
  Bus Creator3/1 -> Data(2B)/1
  Data_0(2B)/1 -> Bus Selector1/1
  Data_1(2B)/1 -> Bus Selector/1
  Name2/1 -> Bus Creator3/1  "b15"
  Name1/1 -> Bus Creator3/2  "b14"
  Name7/1 -> Bus Creator3/3  "b13"
  Name3/1 -> Bus Creator3/4  "b12"
  Name4/1 -> Bus Creator3/5  "b11"
  Name5/1 -> Bus Creator3/6  "b10"
  Name6/1 -> Bus Creator3/7  "b09"
  Name8/1 -> Bus Creator3/8  "b08"
  Bus Selector/8 -> Name8/1  "<b00>"
  Bus Selector/7 -> Name6/1  "<b01>"
  Bus Selector/6 -> Name5/1  "<b02>"
  Bus Selector/5 -> Name4/1  "<b03>"
  Bus Selector/4 -> Name3/1  "<b04>"
  Bus Selector/3 -> Name7/1  "<b05>"
  Bus Selector/2 -> Name1/1  "<b06>"
  Bus Selector/1 -> Name2/1  "<b07>"
  Bus Selector1/8 -> Bus Creator3/16  "<b00>"
  Bus Selector1/2 -> Bus Creator3/10  "<b06>"
  Bus Selector1/7 -> Bus Creator3/15  "<b01>"
  Bus Selector1/6 -> Bus Creator3/14  "<b02>"
  Bus Selector1/4 -> Bus Creator3/12  "<b04>"
  Bus Selector1/5 -> Bus Creator3/13  "<b03>"
  Bus Selector1/1 -> Bus Creator3/9  "<b07>"
  Bus Selector1/3 -> Bus Creator3/11  "<b05>"

== system Computer/Instruction_OR ==
  note: Word_Or
  A(2B) : Inport
  B(2B) : Inport  Port=2
  Bus Creator : BusCreator  Inputs=16
  Bus Selector : BusSelector  OutputSignals=b15,b14,b13,b12,b11,b10,b09,b08,b07,b06,b05,b04,b03,b02,b01,b00
  Bus Selector1 : BusSelector  OutputSignals=b15,b14,b13,b12,b11,b10,b09,b08,b07,b06,b05,b04,b03,b02,b01,b00
  Logical Operator{,1..15} (16 alike) : Logic  Operator=OR  IconShape=distinctive  AllPortsSameDT=off  OutDataTypeStr=boolean
  A||B(2B) : Outport  OutputWhenDisabled=reset
  wires:
  Logical Operator7/1 -> Bus Creator/8  "b08"
  Logical Operator6/1 -> Bus Creator/7  "b09"
  Logical Operator5/1 -> Bus Creator/6  "b10"
  Logical Operator3/1 -> Bus Creator/4  "b12"
  Logical Operator4/1 -> Bus Creator/5  "b11"
  Bus Selector1/8 -> Logical Operator7/2  "<b08>"
  Bus Selector/8 -> Logical Operator7/1  "<b08>"
  Bus Selector1/7 -> Logical Operator6/2  "<b09>"
  Bus Selector/7 -> Logical Operator6/1  "<b09>"
  Bus Selector1/6 -> Logical Operator5/2  "<b10>"
  Bus Selector/6 -> Logical Operator5/1  "<b10>"
  Bus Selector1/5 -> Logical Operator4/2  "<b11>"
  Bus Selector/5 -> Logical Operator4/1  "<b11>"
  Bus Selector1/4 -> Logical Operator3/2  "<b12>"
  Bus Selector/4 -> Logical Operator3/1  "<b12>"
  Bus Selector/3 -> Logical Operator2/1  "<b13>"
  Bus Selector1/3 -> Logical Operator2/2  "<b13>"
  Bus Selector1/2 -> Logical Operator1/2  "<b14>"
  Bus Selector/2 -> Logical Operator1/1  "<b14>"
  Bus Selector1/1 -> Logical Operator/2  "<b15>"
  Bus Selector/1 -> Logical Operator/1  "<b15>"
  Logical Operator8/1 -> Bus Creator/9  "b07"
  Logical Operator9/1 -> Bus Creator/10  "b06"
  Logical Operator10/1 -> Bus Creator/11  "b05"
  Logical Operator15/1 -> Bus Creator/16  "b00"
  Logical Operator14/1 -> Bus Creator/15  "b01"
  Logical Operator13/1 -> Bus Creator/14  "b02"
  Logical Operator11/1 -> Bus Creator/12  "b04"
  Logical Operator12/1 -> Bus Creator/13  "b03"
  Bus Selector/10 -> Logical Operator9/1  "<b06>"
  Bus Selector/9 -> Logical Operator8/1  "<b07>"
  Bus Selector/11 -> Logical Operator10/1  "<b05>"
  Bus Selector/12 -> Logical Operator11/1  "<b04>"
  Bus Selector/13 -> Logical Operator12/1  "<b03>"
  Bus Selector/14 -> Logical Operator13/1  "<b02>"
  Bus Selector/15 -> Logical Operator14/1  "<b01>"
  Bus Selector/16 -> Logical Operator15/1  "<b00>"
  Bus Selector1/9 -> Logical Operator8/2  "<b07>"
  Bus Selector1/10 -> Logical Operator9/2  "<b06>"
  Bus Selector1/11 -> Logical Operator10/2  "<b05>"
  Bus Selector1/12 -> Logical Operator11/2  "<b04>"
  Bus Selector1/13 -> Logical Operator12/2  "<b03>"
  Bus Selector1/14 -> Logical Operator13/2  "<b02>"
  Bus Selector1/15 -> Logical Operator14/2  "<b01>"
  Bus Selector1/16 -> Logical Operator15/2  "<b00>"
  Logical Operator2/1 -> Bus Creator/3  "b13"
  Logical Operator1/1 -> Bus Creator/2  "b14"
  Logical Operator/1 -> Bus Creator/1  "b15"
  Bus Creator/1 -> A||B(2B)/1
  B(2B)/1 -> Bus Selector1/1
  A(2B)/1 -> Bus Selector/1
